simulink model "Discrete_FPGA_PID"  (R2022a)
settings: Solver=ode4  StartTime=0.0  StopTime=20  FixedStep=0.001  RelTol=1e-3
values from neighbouring files (symbols this model uses):
  k1 = kp+td/t    (= 1)    [ContinuousPID.m]
  k2 = -kp + t/ti - 2*td/t    [ContinuousPID.m]
  k3 = td/t    (= 0)    [ContinuousPID.m]
settings Model: Creator=David  LastModifiedBy=David

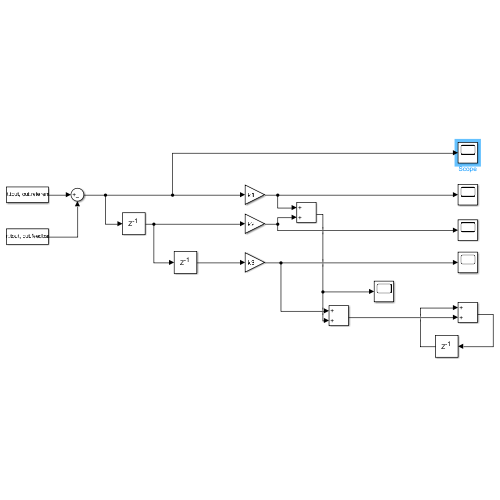
[thumbnail: Simulink's stored preview of the top-level diagram]
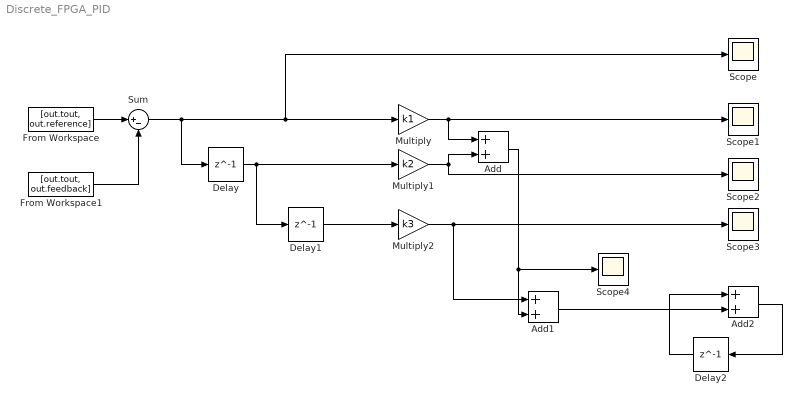
== system Discrete_FPGA_PID ==
  Add : Sum
  Add1 : Sum
  Add2 : Sum
  Delay : Delay  DelayLength=1
  Delay1 : Delay  DelayLength=1
  Delay2 : Delay  DelayLength=1
  From Workspace : FromWorkspace  VariableName=[out.tout, out.reference]
  From Workspace1 : FromWorkspace  VariableName=[out.tout, out.feedback]
  Multiply : Gain  Gain=k1
  Multiply1 : Gain  Gain=k2
  Multiply2 : Gain  Gain=k3
  Scope{,1..4} (5 alike) : Scope
  Sum : Sum  Inputs=|+-
  wires:
  From Workspace/1 -> Sum/1
  From Workspace1/1 -> Sum/2
  Sum/1 -> Delay/1, Scope/1, Multiply/1
  Delay/1 -> Delay1/1, Multiply1/1
  Delay1/1 -> Multiply2/1
  Multiply/1 -> Add/1, Scope1/1
  Multiply1/1 -> Scope2/1, Add/2
  Multiply2/1 -> Scope3/1, Add1/1
  Add1/1 -> Add2/2
  Add2/1 -> Delay2/1
  Delay2/1 -> Add2/1
  Add/1 -> Scope4/1, Add1/2
